simulink library "gravitySubsystem"  (R2021b)
settings: Solver=VariableStepAuto  StartTime=0.0  StopTime=10.0  RelTol=1e-3
libraries: gravityLib x2, conversionsLib x1, aerolibutil x1
settings Model: Creator=mat  LastModifiedBy=mat

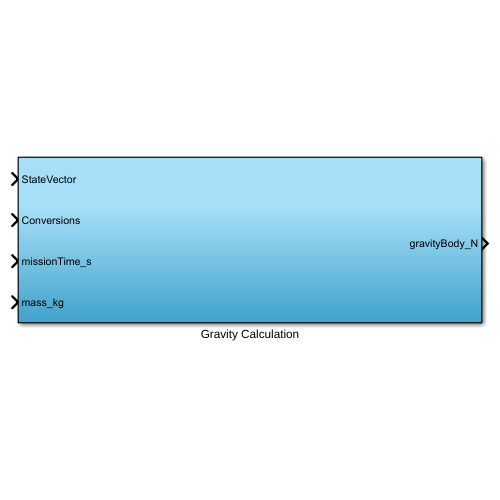
[thumbnail: Simulink's stored preview of the top-level diagram]
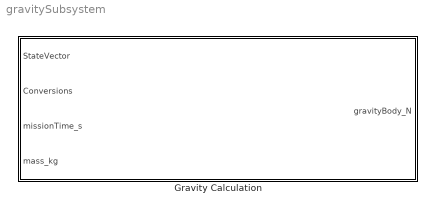
== system gravitySubsystem ==
  Gravity Calculation : Subsystem

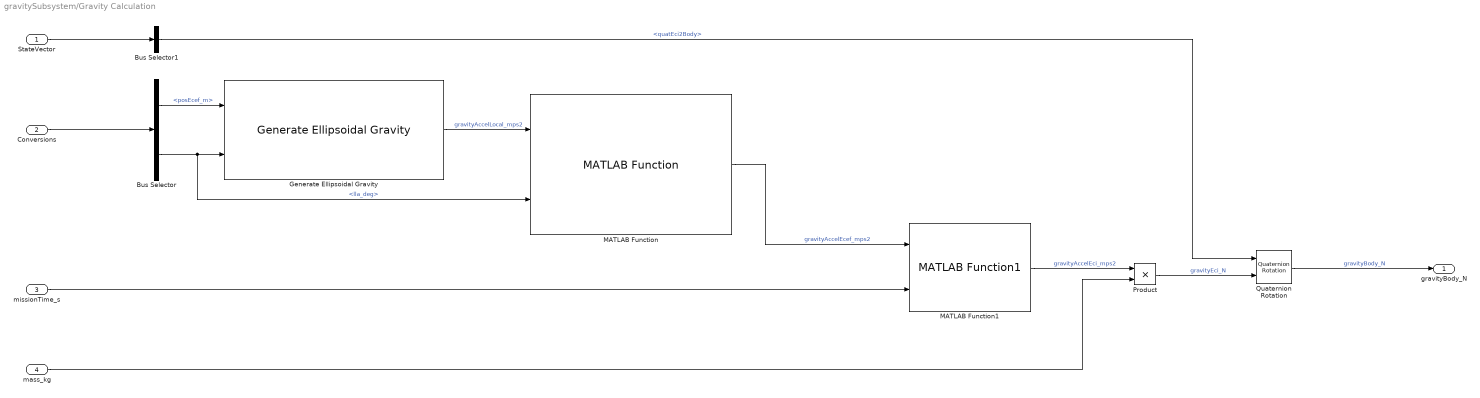
== system gravitySubsystem/Gravity Calculation ==
  StateVector : Inport  OutDataTypeStr=Bus: StateVector_BusType
  Conversions : Inport  Port=2  OutDataTypeStr=Bus: Conversions_BusType
  missionTime_s : Inport  Port=3
  mass_kg : Inport  Port=4
  Bus Selector : BusSelector  OutputSignals=posEcef_m,lla_deg
  Bus Selector1 : BusSelector  OutputSignals=quatEci2Body
  Generate Ellipsoidal Gravity : gravityLib/Generate Ellipsoidal Gravity  SystemSampleTime=-1  VariantActivationTime=update diagram  Latency=0  AutoFrameSizeCalculation=off
  MATLAB Function : gravityLib/MATLAB Function  SystemSampleTime=-1  VariantActivationTime=update diagram  Latency=0  AutoFrameSizeCalculation=off
  MATLAB Function1 : conversionsLib/MATLAB Function1  SystemSampleTime=-1  VariantActivationTime=update diagram  Latency=0  AutoFrameSizeCalculation=off
  Product : Product
  Quaternion Rotation : aerolibutil/Quaternion Rotation
  gravityBody_N : Outport
  wires:
  Quaternion Rotation/1 -> gravityBody_N/1  "gravityBody_N"
  Product/1 -> Quaternion Rotation/2  "gravityEci_N"
  mass_kg/1 -> Product/2
  Bus Selector1/1 -> Quaternion Rotation/1  "<quatEci2Body>"
  StateVector/1 -> Bus Selector1/1
  MATLAB Function1/1 -> Product/1  "gravityAccelEci_mps2"
  missionTime_s/1 -> MATLAB Function1/2
  MATLAB Function/1 -> MATLAB Function1/1  "gravityAccelEcef_mps2"
  Generate Ellipsoidal Gravity/1 -> MATLAB Function/1  "gravityAccelLocal_mps2"
  Bus Selector/2 -> Generate Ellipsoidal Gravity/2, MATLAB Function/2  "<lla_deg>"
  Bus Selector/1 -> Generate Ellipsoidal Gravity/1  "<posEcef_m>"
  Conversions/1 -> Bus Selector/1
